simulink model "fuzzy_logic"  (R2022b)
settings: Solver=VariableStepAuto  StartTime=0.0  StopTime=10.0  RelTol=1e-3
libraries: fuzblock x1
settings Model: Creator=StudentPA  LastModifiedBy=StudentPA

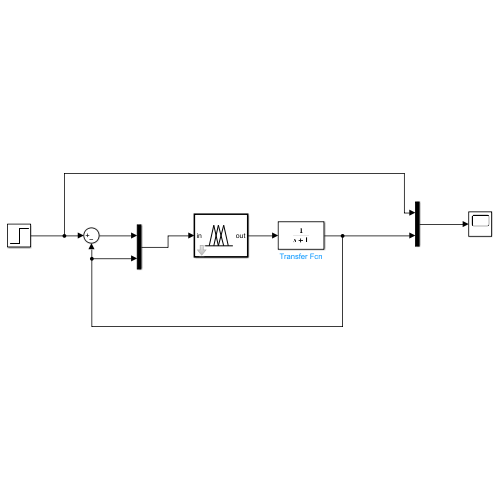
[thumbnail: Simulink's stored preview of the top-level diagram]
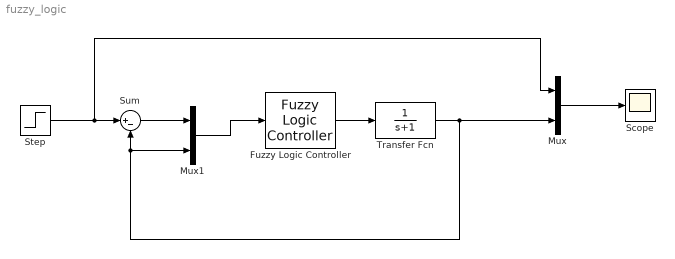
== system fuzzy_logic ==
  Fuzzy Logic Controller : fuzblock/Fuzzy Logic  Controller  FIS=fuzzy_reg  OutputSampleNumber=101  DataType=double  FuzzifiedInputs=off  RuleFiringStrengths=off  RuleOutputs=off  AggregatedOutputs=off  SimulateUsing=Interpreted execution  OutOfRangeInputValueMessage=warning  NoRuleFiredMessage=warning  EmptyOutputFuzzySetMessage=warning
  Mux : Mux  Inputs=2
  Mux1 : Mux  Inputs=2
  Scope : Scope
  Step : Step  SampleTime=0
  Sum : Sum  Inputs=|+-
  Transfer Fcn : TransferFcn  Denominator=[1 1]
  wires:
  Step/1 -> Mux/1, Sum/1
  Transfer Fcn/1 -> Mux1/2, Sum/2, Mux/2
  Mux/1 -> Scope/1
  Fuzzy Logic Controller/1 -> Transfer Fcn/1
  Sum/1 -> Mux1/1
  Mux1/1 -> Fuzzy Logic Controller/1
